simulink model "DiscreteSystemSimulation"  (R2022b)
settings: Solver=FixedStepAuto  StartTime=0.0  StopTime=50  RelTol=1e-3
settings Model: Creator=lang lang  LastModifiedBy=lang lang

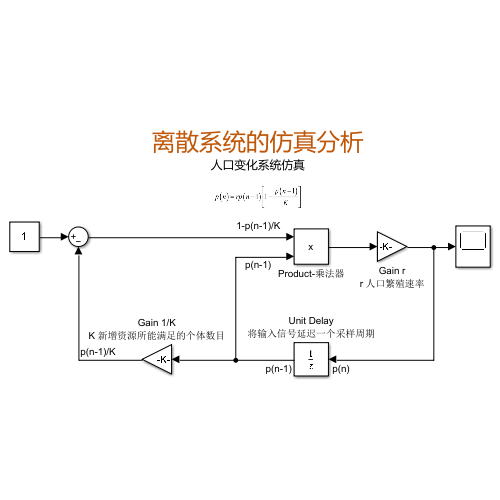
[thumbnail: Simulink's stored preview of the top-level diagram]
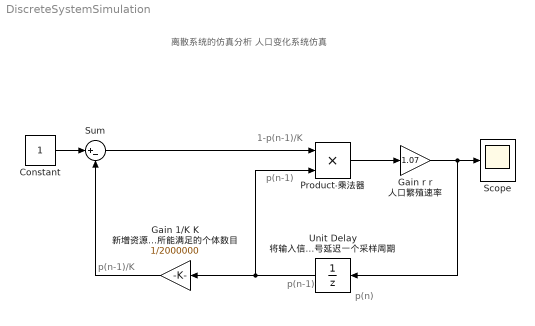
== system DiscreteSystemSimulation ==
  note: p(n-1)
  note: 离散系统的仿真分析
      | 人口变化系统仿真
  note: p(n)
  note: p(n-1)/K
  note: 1-p(n-1)/K
  note: p(n-1)
  Constant : Constant
  Gain 1/K K 新增资源所能满足的个体数目 : Gain  Gain=1/2000000
  Gain r r 人口繁殖速率 : Gain  Gain=1.07
  Product-乘法器 : Product
  Scope : Scope
  Sum : Sum  Inputs=|+-
  Unit Delay 将输入信号延迟一个采样周期 : UnitDelay  InitialCondition=500000  SampleTime=-1  HasFrameUpgradeWarning=on
  wires:
  Product-乘法器/1 -> Gain r r 人口繁殖速率/1
  Unit Delay 将输入信号延迟一个采样周期/1 -> Product-乘法器/2, Gain 1/K K 新增资源所能满足的个体数目/1
  Gain 1/K K 新增资源所能满足的个体数目/1 -> Sum/2
  Constant/1 -> Sum/1
  Sum/1 -> Product-乘法器/1
  Gain r r 人口繁殖速率/1 -> Unit Delay 将输入信号延迟一个采样周期/1, Scope/1
